simulink model "f280049C_DCDC_Buck_PCMC"  (R2021b)
settings: Solver=FixedStepDiscrete  StartTime=0.0  StopTime=Inf  RelTol=1e-3  EnableMultiTasking=on
undefined symbols (not defined in the file or in its folder): codertarget, EALLOW, EDIS, GPTRIP1SEL, TZ1
libraries: c2837xDlib x2, simulink x2, c280xlib x2, c2802xlib x2, c28004xlib x2, c2000lib x1, demo_controls x1, idelinklib_common x1, c2806xlib x1
settings Model: ExtModeTrigDuration=8  Creator=The MathWorks, Inc.  LastModifiedBy=The MathWorks, Inc.
settings SolverCC: AlgebraicLoopSolver=TrustRegion
settings DataIOCC: LimitDataPoints=on  SaveFormat=Array  SaveOutput=off  SaveTime=off  ReturnWorkspaceOutputs=off
settings OptimizationCC: DefaultParameterBehavior=Inlined  DefaultUnderspecifiedDataType=single  UseSpecifiedMinMax=on  MemcpyThreshold=512  NoFixptDivByZeroProtection=on  EfficientFloat2IntCast=on  LifeSpan=inf  MaxStackSize=1024  DenormalBehavior=FlushToZero  EfficientTunableParamExpr=on
settings DebuggingCC: SolverPrmCheckMsg=warning  InheritedTsInSrcMsg=none  MultiTaskDSMMsg=none  ParameterPrecisionLossMsg=none  SFUnexpectedBacktrackingDiag=warning  SFNoUnconditionalDefaultTransitionDiag=warning  SFExecutionAtInitializationDiag=none  SFMachineParentedDataDiag=warning  ArithmeticOperatorsInVariantConditions=warning
settings HardwareCC: ProdBitPerChar=16  ProdBitPerInt=16  ProdBitPerPointer=32  ProdBitPerSizeT=32  ProdBitPerPtrDiffT=32  ProdLargestAtomicInteger=Integer  ProdLargestAtomicFloat=None  ProdWordSize=16  ProdHWDeviceType=Texas Instruments->C2000
settings ModelReferenceCC: PropagateSignalLabelsOutOfModel=off
settings SFSimCC: SimUseLocalCustomCode=off  MATLABDynamicMemAlloc=off  CustomCodeUndefinedFunction=UseInterfaceOnly
settings RTWCC: Description=Embedded Coder  SystemTargetFile=ert.tlc  HardwareBoard=TI Piccolo F280049C LaunchPad  TemplateMakefile=ert_default_tmf  GenerateReport=on  RTWUseLocalCustomCode=off  Toolchain=Texas Instruments Code Composer Studio (C2000)  BuildConfiguration=Specify  IncludeHyperlinkInReport=on  GenerateTraceInfo=on  GenerateTraceReport=on  GenerateTraceReportSl=on  GenerateTraceReportSf=on  GenerateTraceReportEml=on  GenerateCodeMetricsReport=on  GenerateCodeReplacementReport=on
settings CodeAppCC: IgnoreCustomStorageClasses=off  CustomSymbolStrType=$N$R$M  StateflowObjectComments=on
settings ERTTargetCC: CodeReplacementLibrary=TI C28x  IncludeMdlTerminateFcn=off  ExtModeStaticAllocSize=5000  MemSecPackage=tic2000demospkg

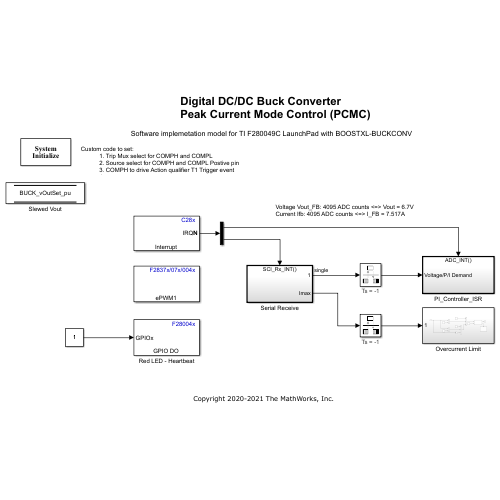
[thumbnail: Simulink's stored preview of the top-level diagram]
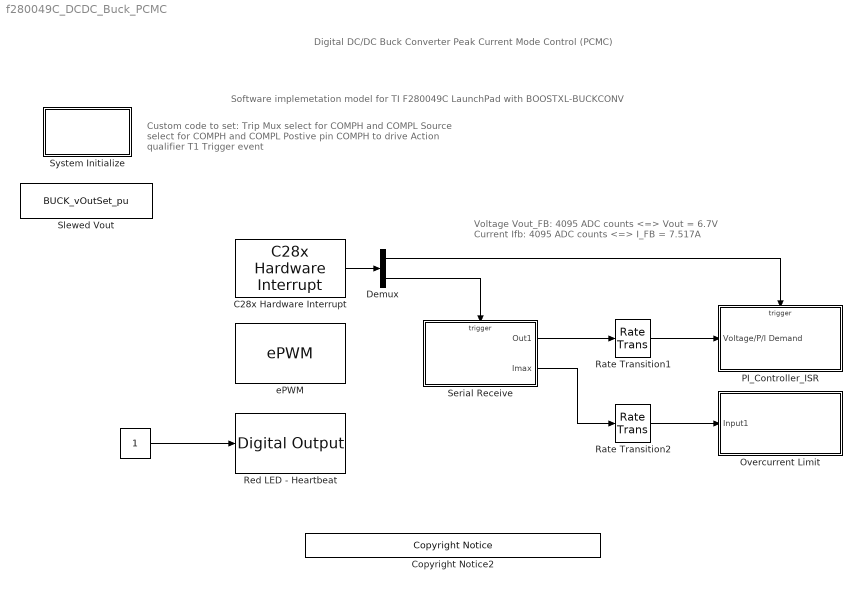
== system f280049C_DCDC_Buck_PCMC ==
  note: Voltage Vout_FB: 4095 ADC counts <=> Vout = 6.7V
      | Current Ifb: 4095 ADC counts <=> I_FB = 7.517A
  note: Digital DC/DC Buck Converter
      | Peak Current Mode Control (PCMC)
  note: Software implemetation model for TI F280049C LaunchPad with BOOSTXL-BUCKCONV
  note: Custom code to set:
      | Trip Mux select for COMPH and COMPL
      | Source select for COMPH and COMPL Postive pin
      | COMPH to drive Action qualifier T1 Trigger event
  "   " : Constant  OutDataTypeStr=uint16  SampleTime=0.1
  C28x Hardware Interrupt : c2000lib/Scheduling/C28x Hardware Interrupt  irqnumbers=[1 9]  pienumbers=[3 1]  irqpriorities=[30 50]  irqpreempts=[0 1]  showinput=off  dspchiptype=C280X
      settings: SourceProductBaseCode=TIC2000
  Copyright Notice2 : demo_controls/Copyright Notice  year=2020  prod=tic2000
      settings: SourceProductBaseCode=ME
  Demux : Demux  Outputs=2
  Overcurrent Limit : Subsystem  Priority=1
  PI_Controller_ISR : Subsystem
      settings: RTWSystemCode=Nonreusable function
  Rate Transition1 : RateTransition  Integrity=off
      settings: AttributesFormatString=Ts = %<OutPortSampleTime>
  Rate Transition2 : RateTransition  Integrity=off
      settings: AttributesFormatString=Ts = %<OutPortSampleTime>
  Red LED - Heartbeat : c28004xlib/Digital Output  GPIO_Number=GPIO16~GPIO23  GPIO_Bit0=off  GPIO_BIT0_Toggle=off  GPIO_Bit1=off  GPIO_BIT1_Toggle=off  GPIO_Bit2=off  GPIO_BIT2_Toggle=off  GPIO_Bit3=off  GPIO_BIT3_Toggle=off  GPIO_Bit4=off  GPIO_BIT4_Toggle=off  GPIO_Bit5=off  GPIO_BIT5_Toggle=off  GPIO_Bit6=off  GPIO_BIT6_Toggle=off  GPIO_Bit7=on  GPIO_BIT7_Toggle=on
      settings: SourceProductBaseCode=TIC2000
  Serial Receive : Subsystem  SystemSampleTime=1e-3
  Slewed Vout : DataStoreMemory  DataStoreName=BUCK_vOutSet_pu  EmbeddedSignalClassName=tic2000demospkg.Signal  ShowAdditionalParam=off  OutDataTypeStr=single
  System Initialize : Subsystem  mask(System Initialize){ShowInLibBrowser=0}
      mask prompts: ShowInLibBrowser "Simulink:masks:CustCodeMaskParam1_MP"
      settings: CopyFcn=cccopyfcn(gcb)  OpenFcn=ccopenfcn('System Initialize Function')
      mask Help: eval('feval(''rtwprivate'',''rtwhelpview'',''rtw_sys_initialize_block'')');
      mask Display: disp('System\nInitialize');
  ePWM : c2802xlib/ePWM  Priority=2  PwmType=C2000_Type4  useModule=ePWM1  ePWMxLINKTBPRD=Not Linked  periodUnits=Clock cycles  timerSource=Specify via dialog  timerPeriod_clk=499  timerPeriod_sec=0.0001  tbshadow=Counter equals to zero  countingMode=Up  phaseActiveEnable=Disable  phaseDirection=Count down after sync  phaseActive=0  synchronizationEnable=off  dcaevt1Sync=off  dcbevt1Sync=off  synchronizationOption=Disable  perSynchronizationOption=Counter equals to period (CTR=PRD)  clockPrescale=1  HSclockPrescale=1  enswap=off  ePWMxAStatus=on  ePWMxAactionLogic1=Set  ePWMxAactionLogic2=Do nothing  ePWMxAactionLogic3=Do nothing  ePWMxAactionLogic4=Set  ePWMxAactionLogic5=Do nothing  ePWMxAactionLogic6=Do nothing  ePWMxACSFenable=off  ePWMxACSFvalue=Forcing disable  ePWMxASFreload=Zero  ePWMxBStatus=off  ePWMxBactionLogic1=Do nothing  ePWMxBactionLogic2=Do nothing  ePWMxBactionLogic3=Do nothing  ePWMxBactionLogic4=Do nothing  ePWMxBactionLogic5=Do nothing  ePWMxBactionLogic6=Set  ePWMxBCSFenable=off  ePWMxBCSFvalue=Forcing disable  ePWMxBSFreload=Zero  ePWNxBOutWay=off  ePWMxLINKCMPA=Not Linked  CMPAUnits=Clock cycles  CMPASource=Specify via dialog  CMPAValue_per=50  CMPAValue_clk=0  enCMPAshadow=Counter equals to period (CTR=PRD)  ePWMxLINKCMPB=Not Linked  CMPBUnits=Clock cycles  CMPBSource=Specify via dialog  CMPBValue_per=50  CMPBValue_clk=315  enCMPBshadow=Counter equals to zero (CTR=Zero)  ePWMxLINKCMPC=Not Linked  CMPCUnits=Clock cycles  CMPCSource=Specify via dialog  CMPCValue_per=50  CMPCValue_clk=32000  enCMPCshadow=Counter equals to zero (CTR=Zero)  ePWMxLINKCMPD=Not Linked  CMPDUnits=Clock cycles  CMPDSource=Specify via dialog  CMPDValue_per=50  CMPDValue_clk=32000  enCMPDshadow=Counter equals to zero (CTR=Zero)  enableDBePWMxA=on  enableDBePWMxB=on  enhalfcycle=off  DBpolarity=Active high complementary (AHC)  DBedgeDelay=Positive  DBSource_ePWMxA=ePWMxA  DBSource_ePWMxB=ePWMxA  DBPeriodUnits=Clock cycles  DBperiodSource=Specify via dialog  REDperiod=15  FEDperiod=15  REDperiod_sec=0  FEDperiod_sec=0  LoadModeDBRED=Immediate without using shadow  LoadModeDBFED=Immediate without using shadow  adcstartModuleA=on  adcrequestEventA=First event  adcstartEventA=Digital Compare Module A Event 1 start of conversion (DCAEVT1.soc)  adcstartEventA_type2=Counter is incrementing and equals to the compare B register (CTRU=CMPB)  adcstartModuleB=off  adcrequestEventB=First event  adcstartEventB=Counter equals to zero (CTR=Zero)  adcstartEventB_type2=Counter equals to zero (CTR=Zero)  intEn=off  intPrd=First event  intSel=Counter equals to zero (CTR=Zero)  intSel_type2=Counter equals to zero (CTR=Zero)  hrpe=off  enHRPWM=off  HRPWM_LoadMode=Counter equals to period (CTR=PRD)  HRPWM_CTLMode=Duty or Period control mode  HRPWM_EDGMode=Both edge  hrpeb=off  enHRPWMB=off  HRPWM_LoadModeB=Counter equals to zero (CTR=ZERO)  HRPWM_CTLModeB=Duty or Period control mode  HRPWM_EDGModeB=Both edge  enHRDBRED=off  enHRDBFED=off  enSFO=on  enautoconv=on  chopperEnable=off  chopperFrequency=1  chopperFirstwidth=1  chopperDuty=12.5%  tripZonesource=Specify via dialog  tzselOSHT1=off  tzselOSHT2=off  tzselOSHT3=off  tzselOSHDCAEV1=on  tzselOSHDCBEV1=off  tzselCBC1=off  tzselCBC2=off  tzselCBC3=off  tzselCBCDCAEV2=off  tzselCBCDCBEV2=off  tzselOSHT4=off  tzselOSHT5=off  tzselOSHT6=off  tzselCBC4=off  tzselCBC5=off  tzselCBC6=off  enTzOstIntr=off  enTzCbcIntr=off  enTzDCAEVT1Intr=off  enTzDCAEVT2Intr=off  enTzDCBEVT1Intr=off  enTzDCBEVT2Intr=off  ePWMxAforced=Low  ePWMxBforced=No action  DCAEVT1forced=No action  DCBEVT1forced=No action  DCAEVT2forced=No action  DCBEVT2forced=No action  dcah=Trip Zone 1 input (TZ1)  dcal=Trip Zone 2 input (TZ2)  dcbh=Trip Zone 1 input (TZ1)  dcbl=Trip Zone 2 input (TZ2)  dcah_type2=GPTRIP5SEL  dcal_type2=GPTRIP4SEL  dcbh_type2=GPTRIP1SEL/(TZ1)  dcbl_type2=GPTRIP1SEL/(TZ1)  gendcaevt1=DCAL=high and DCAH=don't care  gendcaevt2=DCAH=high and DCAL=don't care  gendcbevt1=Event disabled  gendcbevt2=Event disabled  dcaevt1src=DCAEVT1 with async  dcaevt2src=DCEVTFILT with async  dcbevt1src=DCBEVT1 with sync  dcbevt2src=DCBEVT2 with sync  pulsesel=Counter equals to zero (CTR=Zero)  blankinv=off  blankoffset=494  blankwidth=5  evsrcsel=Filtered version of DCAEVT2 (DCAEVT2FILT)  encape=off
  wires:
  Demux/2 -> Serial Receive/Trigger
  C28x Hardware Interrupt/1 -> Demux/1
  "   "/1 -> Red LED - Heartbeat/1
  Demux/1 -> PI_Controller_ISR/Trigger
  Serial Receive/1(Out1) -> Rate Transition1/1
  Rate Transition1/1 -> PI_Controller_ISR/1(Voltage/P/I Demand)
  Serial Receive/2(Imax) -> Rate Transition2/1
  Rate Transition2/1 -> Overcurrent Limit/1(Input1)

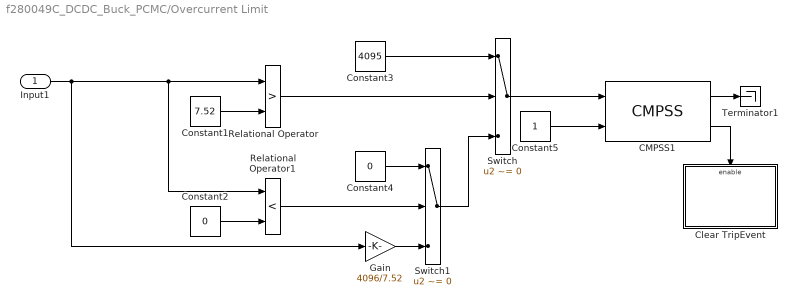
== system f280049C_DCDC_Buck_PCMC/Overcurrent Limit ==
  Input1 : Inport
  CMPSS1 : c2837xDlib/CMPSS  Priority=1  Module=CMPSS1_COMPL  NegativeInput=Internal DAC  DacValueSourceSel=DAC module  DacValueVia=Input port  DACHValue=0  DACLValue=0  RampMaxRefVal=0  RampDecVal=0  RampDelayVal=0  EnableLatchOut=on  EnableLatchClear=on  SampleTime=-1
      settings: SourceProductBaseCode=TIC2000
  Clear TripEvent : Subsystem
  Constant1 : Constant  Value=7.52  OutDataTypeStr=single
  Constant2 : Constant  Value=0  OutDataTypeStr=Inherit: Inherit via back propagation
  Constant3 : Constant  Value=4095  OutDataTypeStr=uint16
  Constant4 : Constant  Value=0  OutDataTypeStr=uint16
  Constant5 : Constant  OutDataTypeStr=uint16
  Gain : Gain  Gain=4096/7.52  OutDataTypeStr=uint16
  Relational Operator : RelationalOperator  Operator=>  OutDataTypeStr=boolean  RndMeth=Nearest
  Relational Operator1 : RelationalOperator  Operator=<  OutDataTypeStr=boolean  RndMeth=Nearest
  Switch : Switch  Criteria=u2 ~= 0  RndMeth=Simplest
  Switch1 : Switch  Criteria=u2 ~= 0  RndMeth=Simplest
  Terminator1 : Terminator
  wires:
  Constant2/1 -> Relational Operator1/2
  Relational Operator/1 -> Switch/2
  Input1/1 -> Relational Operator1/1, Relational Operator/1, Gain/1
  Constant3/1 -> Switch/1
  Switch1/1 -> Switch/3
  Relational Operator1/1 -> Switch1/2
  Constant1/1 -> Relational Operator/2
  Constant4/1 -> Switch1/1
  Gain/1 -> Switch1/3
  CMPSS1/2 -> Clear TripEvent/Enable
  CMPSS1/1 -> Terminator1/1
  Switch/1 -> CMPSS1/1
  Constant5/1 -> CMPSS1/2

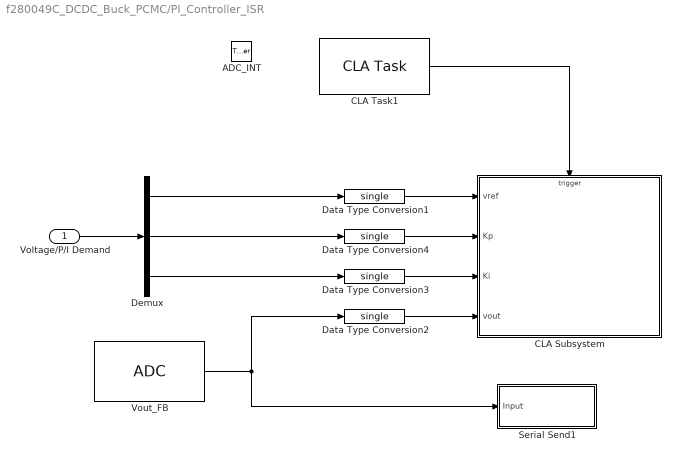
== system f280049C_DCDC_Buck_PCMC/PI_Controller_ISR ==
  Voltage/P/I Demand : Inport
  ADC_INT : TriggerPort  TriggerType=function-call  VariantControl=Variant  PortDimensions=1
  CLA Subsystem : Subsystem  InitFcn=codertarget.registry.registerC28xNonPeripheralBlocks(gcb)  TreatAsAtomicUnit=on  RTWFileName=sample_cla  mask(c28x CLA Subsystem){}
      settings: CopyFcn=codertarget.registry.setC28xCLASubSystem(gcb)  OpenFcn=open_system(gcbh,'force')  RTWSystemCode=Nonreusable function  RTWFileNameOpts=User specified  FunctionWithSeparateData=on  RTWMemSecFuncInitTerm=C28xFunction  RTWMemSecFuncExecute=ClaFunction  RTWMemSecDataConstants=Cla1DataRam  RTWMemSecDataInternal=Cla1DataRam  RTWMemSecDataParameters=Cla1DataRam
      mask Display: color('black'); text(0.50, 0.12, 'CLA Subsystem', 'horizontalAlignment','center');
  CLA Task1 : c2806xlib/CLA Task  taskNumber=1  intSource=Software  sampleTime=-1  claType=2  softTrigSelected=1  enableInterrupt=on
      settings: SourceProductBaseCode=TIC2000
  Data Type Conversion{1..4} (4 alike) : DataTypeConversion  OutDataTypeStr=single
  Demux : Demux  Outputs=3
  Serial Send1 : Subsystem
  Vout_FB : c2802xlib/ADC  blkParamProc=C2000_Type5  ADCModule=C  samplingMode=Single sample mode  ADCResolution=12-bit (Single-ended input)  useSOC1=SOC0  useSOC2=SOC0_SOC1  SOCAcquisitionWindow=10  SOCTriggerSource=ePWM1_ADCSOCA  SOCInterruptTrigger=No ADCINT  Ts=-1  dType=uint16  postInterrupt=on  interruptSel=ADCINT1  ADCINTContinuous=off  endma=off  chdma=1  conv1=ADCINA0  conv2=ADCINA0 and ADCINB0  conv1_Type4=ADCIN3  conv2_Type4=ADCIN0 and ADCIN1
  wires:
  Voltage/P/I Demand/1 -> Demux/1
  CLA Task1/1 -> CLA Subsystem/Trigger
  Demux/1 -> Data Type Conversion1/1
  Vout_FB/1 -> Serial Send1/1(Input), Data Type Conversion2/1
  Demux/3 -> Data Type Conversion3/1
  Data Type Conversion2/1 -> CLA Subsystem/4(vout)
  Demux/2 -> Data Type Conversion4/1
  Data Type Conversion1/1 -> CLA Subsystem/1(vref)
  Data Type Conversion3/1 -> CLA Subsystem/3(Ki)
  Data Type Conversion4/1 -> CLA Subsystem/2(Kp)

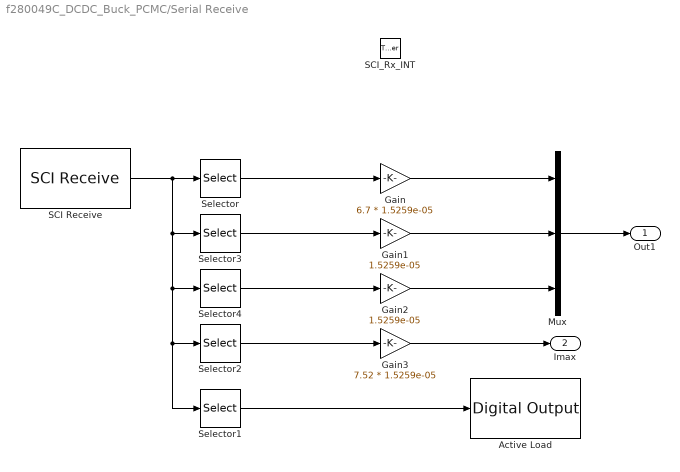
== system f280049C_DCDC_Buck_PCMC/Serial Receive ==
  SCI_Rx_INT : TriggerPort  TriggerType=function-call  VariantControl=Variant
  Active Load : c28004xlib/Digital Output  GPIO_Number=GPIO0~GPIO7  GPIO_Bit0=off  GPIO_BIT0_Toggle=off  GPIO_Bit1=off  GPIO_BIT1_Toggle=off  GPIO_Bit2=on  GPIO_BIT2_Toggle=off  GPIO_Bit3=off  GPIO_BIT3_Toggle=off  GPIO_Bit4=off  GPIO_BIT4_Toggle=off  GPIO_Bit5=off  GPIO_BIT5_Toggle=off  GPIO_Bit6=off  GPIO_BIT6_Toggle=off  GPIO_Bit7=off  GPIO_BIT7_Toggle=off
      settings: SourceProductBaseCode=TIC2000
  Gain : Gain  Gain=6.7 * 1.5259e-05  OutDataTypeStr=single
  Gain1 : Gain  Gain=1.5259e-05  OutDataTypeStr=single
  Gain2 : Gain  Gain=1.5259e-05  OutDataTypeStr=single
  Gain3 : Gain  Gain=7.52 * 1.5259e-05  OutDataTypeStr=single
  Mux : Mux  Inputs=3
  SCI Receive : c280xlib/SCI Receive  sciModule=A  dataHead='S'  dataTail='E'  dataType=uint16  dataDim=5  initValue=0  errOption=Output the last received value  errValue=0  sampleTime=-1  outputStatus=off  postInterrupt=on  numFifo=10
      settings: SourceProductBaseCode=TIC2000
  Selector : Selector  InputPortWidth=5  IndexOptions=Index vector (dialog)  Indices=[1]  OutputSizes=1
  Selector1 : Selector  InputPortWidth=5  IndexOptions=Index vector (dialog)  Indices=[5]  OutputSizes=1
  Selector2 : Selector  InputPortWidth=5  IndexOptions=Index vector (dialog)  Indices=[4]  OutputSizes=1
  Selector3 : Selector  InputPortWidth=5  IndexOptions=Index vector (dialog)  Indices=[2]  OutputSizes=1
  Selector4 : Selector  InputPortWidth=5  IndexOptions=Index vector (dialog)  Indices=[3]  OutputSizes=1
  Out1 : Outport  OutDataTypeStr=single  InitialOutput=[1.999 0.6 0.002]
  Imax : Outport  Port=2  InitialOutput=5.2  VectorParamsAs1DForOutWhenUnconnected=off
  wires:
  SCI Receive/1 -> Selector3/1, Selector4/1, Selector1/1, Selector2/1, Selector/1
  Selector1/1 -> Active Load/1
  Selector/1 -> Gain/1
  Gain/1 -> Mux/1
  Selector2/1 -> Gain3/1
  Selector3/1 -> Gain1/1
  Gain1/1 -> Mux/2
  Gain2/1 -> Mux/3
  Selector4/1 -> Gain2/1
  Mux/1 -> Out1/1
  Gain3/1 -> Imax/1

== system f280049C_DCDC_Buck_PCMC/System Initialize ==

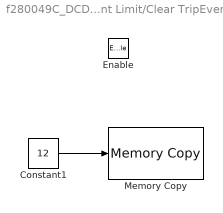
== system f280049C_DCDC_Buck_PCMC/Overcurrent Limit/Clear TripEvent ==
  Enable : EnablePort
  Constant1 : Constant  Value=12  OutDataTypeStr=uint16  SampleTime=-1
  Memory Copy : idelinklib_common/Memory Copy  Priority=2  copyFrom=Input port  copyFromAddressSource=Specify via dialog  copyFromAddress=hex2dec('00001000')  copyFromSrcCode=myVariableSrc  dataTypeFrom=uint16  dataDimensionFrom=1  useOffsetFrom=off  offsetFromSrc=Specify via dialog  offsetFrom=0  strideFrom=1  copyTo=Specified address  copyToAddressSource=Specify via dialog  copyToAddress=hex2dec('00004097')  copyToSrcCode=myVariableDst  dataTypeTo=uint16  useOffsetTo=off  offsetToSrc=Specify via dialog  offsetTo=0  strideTo=1  sampleTime=-1  useInitValue=off  initValueSrc=Specify constant value  initValue=1  initValueSrcCode=myInitValueVariable  useAsMask=off  maskOperator=bitwise AND  useTermValue=off  termValue=1  isRealtimeEnabled=off  emitCCBeforeWrite=on  CCBeforeWrite=EALLOW;  emitCCAfterWrite=on  CCAfterWrite=EDIS;  useDMACopy=off  enableBlockingMode=off
      settings: SourceProductBaseCode=ME
  wires:
  Constant1/1 -> Memory Copy/1

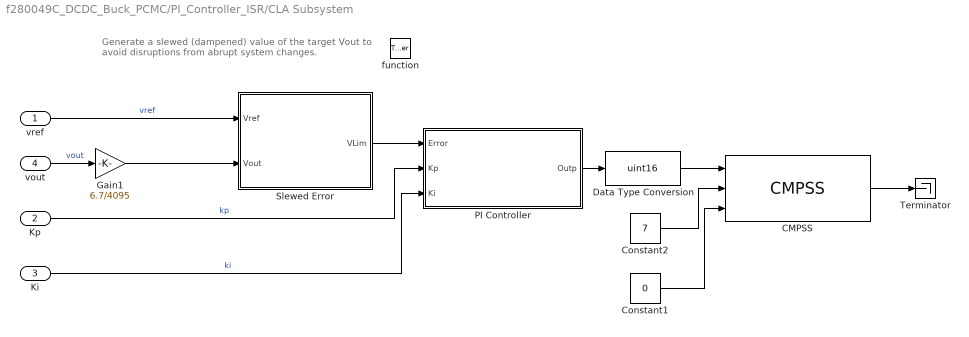
== system f280049C_DCDC_Buck_PCMC/PI_Controller_ISR/CLA Subsystem ==
  note: Generate a slewed (dampened) value of the target Vout to avoid disruptions from abrupt system changes.
  vref : Inport  OutDataTypeStr=single
  Kp : Inport  Port=2  OutDataTypeStr=single
  Ki : Inport  Port=3  OutDataTypeStr=single
  vout : Inport  Port=4  OutDataTypeStr=single
  function : TriggerPort  TriggerType=function-call  VariantControl=Variant
  CMPSS : c2837xDlib/CMPSS  Module=CMPSS1_COMPH  NegativeInput=Internal DAC  DacValueSourceSel=RAMP module  DacValueVia=Input port  DACHValue=0  DACLValue=0  RampMaxRefVal=0  RampDecVal=0  RampDelayVal=0  EnableLatchOut=off  EnableLatchClear=off  SampleTime=0.1
      settings: SourceProductBaseCode=TIC2000
  Constant1 : Constant  Value=0  OutDataTypeStr=uint16  SampleTime=-1
  Constant2 : Constant  Value=7  OutDataTypeStr=uint16  SampleTime=-1
  Data Type Conversion : DataTypeConversion  OutDataTypeStr=uint16
  Gain1 : Gain  Gain=6.7/4095  OutDataTypeStr=single
  PI Controller : Subsystem
  Slewed Error : Subsystem
  Terminator : Terminator
  wires:
  PI Controller/1(Outp) -> Data Type Conversion/1
  Kp/1 -> PI Controller/2(Kp)  "kp"
  Ki/1 -> PI Controller/3(Ki)  "ki"
  CMPSS/1 -> Terminator/1
  Data Type Conversion/1 -> CMPSS/1
  vref/1 -> Slewed Error/1(Vref)  "vref"
  Constant1/1 -> CMPSS/3
  vout/1 -> Gain1/1  "vout"
  Constant2/1 -> CMPSS/2
  Slewed Error/1(VLim) -> PI Controller/1(Error)
  Gain1/1 -> Slewed Error/2(Vout)

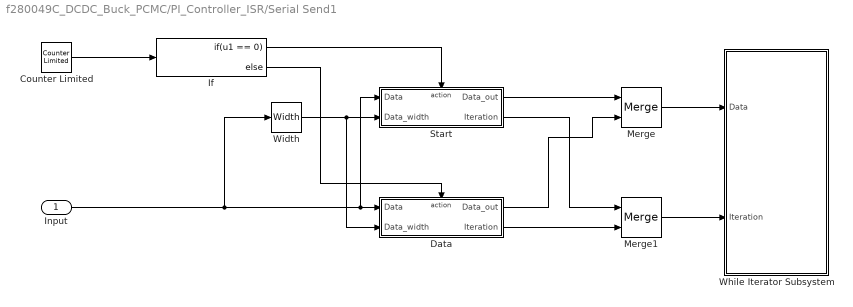
== system f280049C_DCDC_Buck_PCMC/PI_Controller_ISR/Serial Send1 ==
  Input : Inport
  Counter Limited : simulink/Sources/Counter Limited  uplimit=11999  tsamp=-1
  Data : Subsystem  TreatAsAtomicUnit=on
  If : If  IfExpression=u1 == 0
  Merge : Merge
  Merge1 : Merge
  Start : Subsystem  TreatAsAtomicUnit=on
  While Iterator Subsystem : Subsystem  TreatAsAtomicUnit=on
  Width : Width  OutDataTypeMode=All ports same datatype  DataType=uint16
  wires:
  If/1 -> Start/Action
  If/2 -> Data/Action
  Start/1(Data_out) -> Merge/1
  Data/1(Data_out) -> Merge/2
  Merge/1 -> While Iterator Subsystem/1(Data)
  Merge1/1 -> While Iterator Subsystem/2(Iteration)
  Start/2(Iteration) -> Merge1/1
  Data/2(Iteration) -> Merge1/2
  Width/1 -> Data/2(Data_width), Start/2(Data_width)
  Counter Limited/1 -> If/1
  Input/1 -> Width/1, Start/1(Data), Data/1(Data)

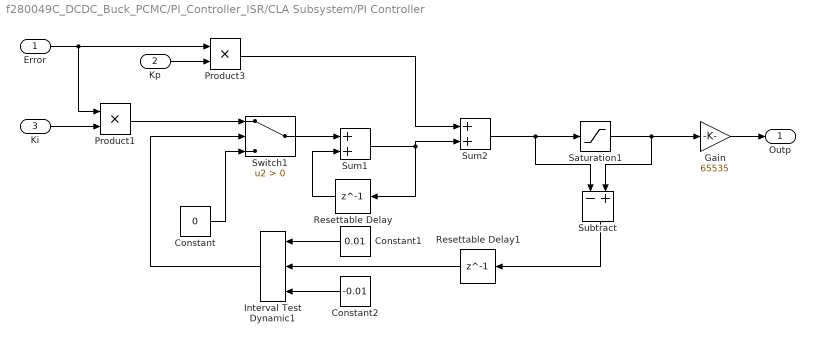
== system f280049C_DCDC_Buck_PCMC/PI_Controller_ISR/CLA Subsystem/PI Controller ==
  Error : Inport
  Kp : Inport  Port=2
  Ki : Inport  Port=3
  Constant : Constant  Value=0  OutDataTypeStr=Inherit: Inherit via back propagation
  Constant1 : Constant  Value=0.01  OutDataTypeStr=Inherit: Inherit via back propagation
  Constant2 : Constant  Value=-0.01  OutDataTypeStr=Inherit: Inherit via back propagation
  Gain : Gain  Gain=65535  OutDataTypeStr=single
  Interval Test Dynamic1 : simulink/Logic and Bit Operations/Interval Test Dynamic  IntervalClosedRight=on  IntervalClosedLeft=on  OutDataTypeStr=boolean
      settings: SourceProductBaseCode=SL
  Product1 : Product
  Product3 : Product
  Resettable Delay : Delay  DelayLength=1
  Resettable Delay1 : Delay  DelayLength=1
  Saturation1 : Saturate  UpperLimit=1.0  LowerLimit=0.0  LinearizeAsGain=off
  Subtract : Sum  Inputs=-+
  Sum1 : Sum
  Sum2 : Sum
  Switch1 : Switch  Criteria=u2 > Threshold
  Outp : Outport  VectorParamsAs1DForOutWhenUnconnected=off
  wires:
  Saturation1/1 -> Subtract/2, Gain/1
  Switch1/1 -> Sum1/1
  Ki/1 -> Product1/2
  Sum1/1 -> Sum2/2, Resettable Delay/1
  Constant/1 -> Switch1/3
  Resettable Delay/1 -> Sum1/2
  Product1/1 -> Switch1/1
  Error/1 -> Product1/1, Product3/1
  Kp/1 -> Product3/2
  Product3/1 -> Sum2/1
  Sum2/1 -> Saturation1/1, Subtract/1
  Gain/1 -> Outp/1
  Subtract/1 -> Resettable Delay1/1
  Interval Test Dynamic1/1 -> Switch1/2
  Constant2/1 -> Interval Test Dynamic1/3
  Constant1/1 -> Interval Test Dynamic1/1
  Resettable Delay1/1 -> Interval Test Dynamic1/2

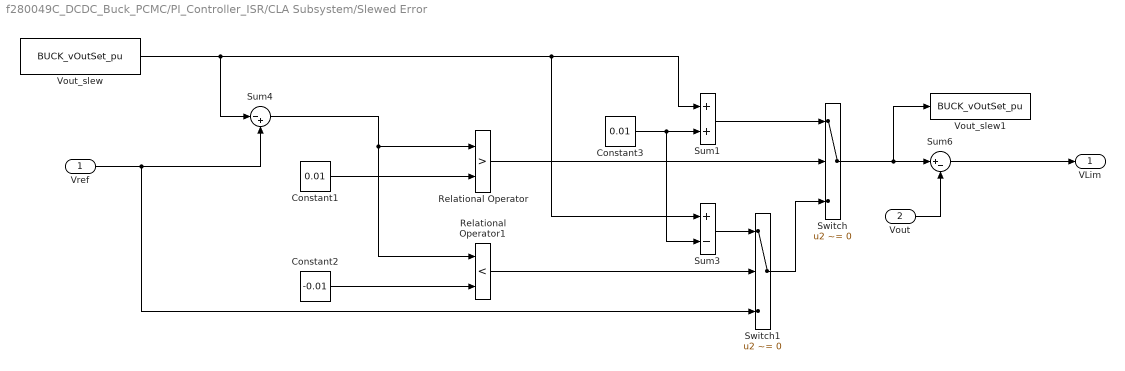
== system f280049C_DCDC_Buck_PCMC/PI_Controller_ISR/CLA Subsystem/Slewed Error ==
  Vref : Inport
  Vout : Inport  Port=2
  Constant1 : Constant  Value=0.01  OutDataTypeStr=Inherit: Inherit via back propagation
  Constant2 : Constant  Value=-0.01  OutDataTypeStr=Inherit: Inherit via back propagation
  Constant3 : Constant  Value=0.01  OutDataTypeStr=Inherit: Inherit via back propagation
  Relational Operator : RelationalOperator  Operator=>  OutDataTypeStr=boolean  RndMeth=Nearest
  Relational Operator1 : RelationalOperator  Operator=<  OutDataTypeStr=boolean  RndMeth=Nearest
  Sum1 : Sum  RndMeth=Simplest  OutDataTypeStr=Inherit: Same as first input
  Sum3 : Sum  Inputs=+-  RndMeth=Simplest  OutDataTypeStr=Inherit: Same as first input
  Sum4 : Sum  Inputs=|-+  RndMeth=Simplest  OutDataTypeStr=Inherit: Same as first input
  Sum6 : Sum  Inputs=|+-  RndMeth=Simplest  OutDataTypeStr=Inherit: Same as first input
  Switch : Switch  Criteria=u2 ~= 0  RndMeth=Simplest
  Switch1 : Switch  Criteria=u2 ~= 0  RndMeth=Simplest
  Vout_slew : DataStoreRead  DataStoreName=BUCK_vOutSet_pu  IndexOptions=Index vector (dialog)  Indices=1  OutputSizes=1
  Vout_slew1 : DataStoreWrite  DataStoreName=BUCK_vOutSet_pu  IndexOptions=Index vector (dialog)  Indices=1  OutputSizes=1
  VLim : Outport  VectorParamsAs1DForOutWhenUnconnected=off
  wires:
  Sum4/1 -> Relational Operator1/1, Relational Operator/1
  Constant3/1 -> Sum3/2, Sum1/2
  Sum3/1 -> Switch1/1
  Relational Operator1/1 -> Switch1/2
  Switch1/1 -> Switch/3
  Sum1/1 -> Switch/1
  Relational Operator/1 -> Switch/2
  Constant1/1 -> Relational Operator/2
  Vref/1 -> Sum4/2, Switch1/3
  Vout_slew/1 -> Sum4/1, Sum3/1, Sum1/1
  Constant2/1 -> Relational Operator1/2
  Switch/1 -> Vout_slew1/1, Sum6/1
  Vout/1 -> Sum6/2
  Sum6/1 -> VLim/1

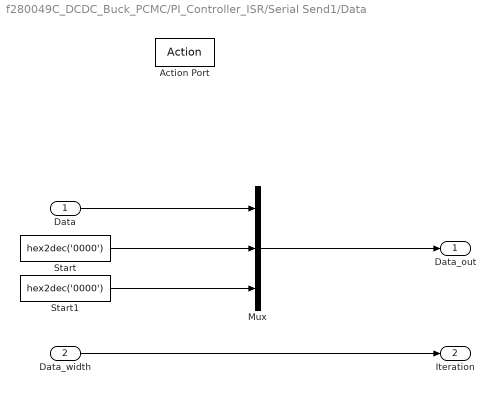
== system f280049C_DCDC_Buck_PCMC/PI_Controller_ISR/Serial Send1/Data ==
  Data : Inport
  Data_width : Inport  Port=2
  Action Port : ActionPort  ActionPortLabel=else
  Mux : Mux  Inputs=3
  Start : Constant  Value=hex2dec('0000')  OutDataTypeStr=uint16
  Start1 : Constant  Value=hex2dec('0000')  OutDataTypeStr=uint16
  Data_out : Outport  VectorParamsAs1DForOutWhenUnconnected=off
  Iteration : Outport  Port=2  VectorParamsAs1DForOutWhenUnconnected=off
  wires:
  Start/1 -> Mux/2
  Mux/1 -> Data_out/1
  Data/1 -> Mux/1
  Data_width/1 -> Iteration/1
  Start1/1 -> Mux/3

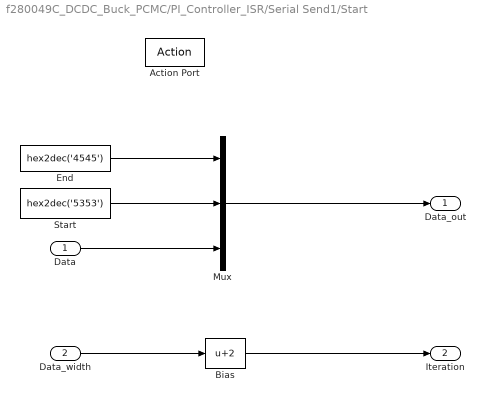
== system f280049C_DCDC_Buck_PCMC/PI_Controller_ISR/Serial Send1/Start ==
  Data : Inport
  Data_width : Inport  Port=2
  Action Port : ActionPort  ActionPortLabel=if(u1 == 0)
  Bias : Bias  Bias=2
  End : Constant  Value=hex2dec('4545')  OutDataTypeStr=uint16
  Mux : Mux  Inputs=3
  Start : Constant  Value=hex2dec('5353')  OutDataTypeStr=uint16
  Data_out : Outport  VectorParamsAs1DForOutWhenUnconnected=off
  Iteration : Outport  Port=2  VectorParamsAs1DForOutWhenUnconnected=off
  wires:
  Start/1 -> Mux/2
  Mux/1 -> Data_out/1
  Data_width/1 -> Bias/1
  Bias/1 -> Iteration/1
  Data/1 -> Mux/3
  End/1 -> Mux/1

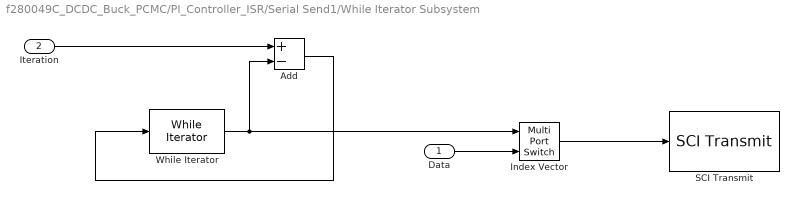
== system f280049C_DCDC_Buck_PCMC/PI_Controller_ISR/Serial Send1/While Iterator Subsystem ==
  Data : Inport
  Iteration : Inport  Port=2
  Add : Sum  Inputs=+-  OutDataTypeStr=Inherit: Same as first input
  Index Vector : MultiPortSwitch  Inputs=1
  SCI Transmit : c280xlib/SCI Transmit  sciModule=A  dataHead=''  dataTail=''  postInterrupt=off  numFifo=1
  While Iterator : WhileIterator  MaxIters=-1  WhileBlockType=do-while  ShowIterationPort=on  OutputDataType=int16
  wires:
  Iteration/1 -> Add/1
  Add/1 -> While Iterator/1
  Index Vector/1 -> SCI Transmit/1
  Data/1 -> Index Vector/2
  While Iterator/1 -> Index Vector/1, Add/2
